simulink model "StateDiagram1"  (R2025b)
settings: Solver=VariableStepAuto  StartTime=0.0  StopTime=Inf  RelTol=1e-3
settings Model: Creator=Soochan Kim  LastModifiedBy=Soochan Kim
settings OptimizationCC: BlockReduction=off  ConditionallyExecuteInputs=off  DefaultParameterBehavior=Inlined
settings DebuggingCC: AlgebraicLoopMsg=error
settings HardwareCC: ProdBitPerPointer=32.0  ProdBitPerSizeT=32.0  ProdBitPerPtrDiffT=32.0  ProdLargestAtomicFloat=None  ProdIntDivRoundTo=Undefined  ProdEndianess=Unspecified  ProdWordSize=32.0  ProdHWDeviceType=ASIC/FPGA->ASIC/FPGA  TargetBitPerPointer=64.0  TargetBitPerSizeT=64.0  TargetBitPerPtrDiffT=64.0  TargetLongLongMode=on  TargetIntDivRoundTo=Zero  TargetEndianess=LittleEndian  TargetWordSize=64.0  TargetHWDeviceType=Custom Processor->MATLAB Host Computer  ProdEqTarget=off

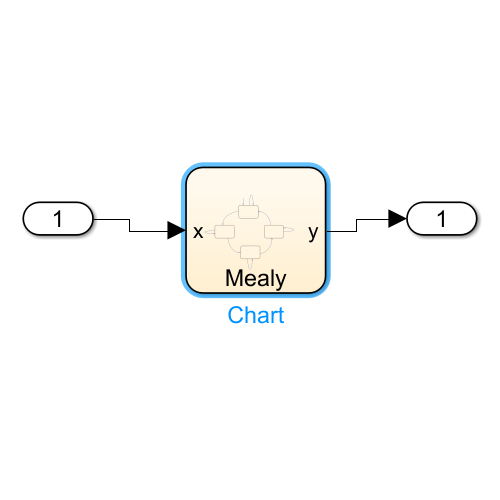
[thumbnail: Simulink's stored preview of the top-level diagram]
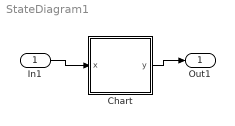
== system StateDiagram1 ==
  In1 : Inport  OutDataTypeStr=boolean
  Chart : Stateflow chart  TreatAsAtomicUnit=on
  Out1 : Outport  VectorParamsAs1DForOutWhenUnconnected=off
  wires:
  In1/1 -> Chart/1(x)
  Chart/1(y) -> Out1/1

== stateflow chart StateDiagram1/Chart ==
  settings: updateMethod=DISCRETE  stateMachineType=MEALY_MACHINE  executeAtInitialization=1
  state S0
  state S02
  state S01
  state S03
  S0 -> S0 [order 2] : [x==0]{y=false}
  (default) -> S0
  S01 -> S0 [order 2] : [x==1]{y=true}
  S0 -> S02 [order 1] : [x==1]{y=false}
  S01 -> S01 [order 1] : [x==0]{y=false}
  S02 -> S02 [order 2] : [x==1]{y=false}
  S02 -> S03 [order 1] : [x==0]{y=false}
  S03 -> S01 [order 1] : [x==0]{y=false }
  S03 -> S03 [order 2] : [x==1]{y=false}
  data: x input boolean; y output boolean
